simulink model "modello_completo_simulink2019b"  (R2019b)
settings: Solver=VariableStepAuto  StartTime=0.0  StopTime=30  RelTol=1e-3
undefined symbols (not defined in the file): a, a1, a2, AHRS_bias, AHRS_sample_time, AHRS_var, alpha1, alpha2, c, current, D, dead_zone_limit, DiscIntNeverNeededParam, DVL_sample_t, DVL_var1, DVL_var2, DVL_var3, gps_sample_t, H, IMU_sample_time, initial, INSP, Ki_bodypos1, Ki_bodypos2, Ki_bodypos3, Ki_bodypos4, Ki_bodypos5, Ki_depth1, Ki_depth2, Ki_depth3, Ki_depth4, Ki_depth5, Ki_latvel1, Ki_latvel2, Ki_latvel3, Ki_latvel4, Ki_latvel5, Ki_P1, Ki_P2, Ki_P3, Ki_P4, Ki_P5, Ki_R1, Ki_R2, Ki_R3, Ki_R4, Ki_R5, Ki_rel_or1, Ki_rel_or2, Ki_rel_or3, Ki_rel_or4, Ki_rel_or5, Ki_reldist1, Ki_reldist2, Ki_reldist3, Ki_reldist4, Ki_reldist5, Ki_surge1, Ki_surge2, Ki_surge3 ... (+66)
libraries: simulink x3
(part 5 of 5)

== matlab function modello_completo_simulink2019b/Vehicle Model/Thrusters/T/Thruster 7/MATLAB Function ==
  data: n input; T output; V input; D parameter; omega parameter; a1 parameter; a2 parameter; alpha1 parameter; alpha2 parameter
function T = thrusterModel(n, V, D, omega, a1, a2, alpha1, alpha2)

Va = (1-omega) * V;     % Advancement velocity at the propeller
J0 = Va/(n*D);          % Advancement Coefficient

if J0 > -alpha1/alpha2  % Out of linearity domain (right side)
    T = 0;              % A null generated thrust is assumed
    
elseif J0 < 0           % Out of linearity domain (left side)
    T = a1*abs(n)*n;    % Bollard thrust is assumed

else                    % Within the linearity domain
    T = a1*abs(n)*n - a2*abs(n)*V;
end

== matlab function modello_completo_simulink2019b/Vehicle Model/Model Vehicle/MATLAB Function ==
  data: coord_pylon input; eta input; eta_ecef output
function eta_ecef = nedToEcef(coord_pylon, eta)

    coder.extrinsic('wgs84Ellipsoid');

    coder.extrinsic('ned2geodetic');
    
    eta_pos = eta(1:6);
    wgs84 = wgs84Ellipsoid('meter'); %TODO verificare che esprima le coordinate nello stesso modo dell'ECEF dato in missionB.m
    [eta_pos(1), eta_pos(2)] = ned2geodetic(eta(1), eta(2), eta(3), coord_pylon(1), coord_pylon(2), coord_pylon(3), wgs84,'degrees');
    
    eta_pos(3) = eta(3);
    eta_pos(4:6) = eta_pos(4:6);
    
    eta_ecef = eta_pos;
    
end

== matlab function modello_completo_simulink2019b/Vehicle Model/MATLAB Function ==
  data: eta input; ni_c output; current input
function ni_c = current_ned2body(eta, current)
    eta2 = eta(4:6)*pi/180;     % eta2 espresso in radianti
    ni_c = Jac(eta2)'*current;
end

== matlab function modello_completo_simulink2019b/Vehicle Model/Thrusters/T/MATLAB Function ==
  data: ni input; v_th output
function v_th = thrusters(ni)
p1 = [-0.35 -0.25 0]';
p2 = [-0.35 0.25 0]';
p3 = [-0.25 -0.35 0]';
p4 = [0.25 0.35 0]';
p5 = [-0.25 -0.25 -0.19]';
p6 = [-0.25 0.25 -0.19]';
p7 = [0.25 0 -0.19]';

t1 = [1 0 0]';
t2 = t1;
t3 = [0 1 0]';
t4 = -t3;
t5 = [0 0 1]';
t6 = t5;
t7 = t5;

v_lin = ni(1:3);
v_ang = ni(4:6);

vp1 = v_lin + cross(v_ang, p1);
vp2 = v_lin + cross(v_ang, p2);
vp3 = v_lin + cross(v_ang, p3);
vp4 = v_lin + cross(v_ang, p4);
vp5 = v_lin + cross(v_ang, p5);
vp6 = v_lin + cross(v_ang, p6);
vp7 = v_lin + cross(v_ang, p7);

v1 = vp1'*t1;
v2 = vp2'*t2;
v3 = vp3'*t3;
v4 = vp4'*t4;
v5 = vp5'*t5;
v6 = vp6'*t6;
v7 = vp7'*t7;

v_th = [ v1 v2 v3 v4 v5 v6 v7]';
end

== matlab function modello_completo_simulink2019b/Navigation1/Geodetic to NED/MATLAB Function2 ==
  data: GPS_geodetic input; GPS_flag input; GPS_NED output; depth input; pylonCenter parameter
function GPS_NED = Geo2NED(GPS_geodetic, GPS_flag, depth, pylonCenter)

% Funzione che trasforma le coordinate dal sistema di riferimento geodetico
% ad un sistema NED con origine in corrispondenza del centro del pilone.

%% GPS non funzionante
if GPS_flag == 0            
    GPS_NED = [0;0;0];
    return
end

%% Variabili
phi = GPS_geodetic(1);                  % Coordinate geodetiche in radianti                     
lambda = GPS_geodetic(2);  
h = -depth;

phi_pyl = pylonCenter(1) * pi/180;      % Origine del sistema NED in coordinate geodetiche
lambda_pyl = pylonCenter(2) * pi/180;

%% Trasformazione coordinate
coder.extrinsic('wgs84Ellipsoid');
coder.extrinsic('geodetic2ned');
    
[x_gps2, y_gps2, z_gps2] = geodetic2ned(phi, lambda, -depth, phi_pyl, lambda_pyl, 0, wgs84Ellipsoid, 'radians');
eta_NED_GPS = [x_gps2; y_gps2];

GPS_NED = zeros(3,1);
GPS_NED(1) = eta_NED_GPS(1);            % Coordiante NED in radianti
GPS_NED(2) = eta_NED_GPS(2);
GPS_NED(3) = GPS_flag;

== matlab function modello_completo_simulink2019b/Vehicle Model/Thrusters/saturation_tau ==
  data: tau input; tau_sat output; eta input
function tau_sat = sat_tau(tau, eta)
    tau_sat = [0;0;0;0;0;0];
    tau_sat = tau;

    if eta(3) < 0.1 %semiasse c
        tau_sat(3) = 0;
    end
    
end

== matlab function modello_completo_simulink2019b/Navigation1/MATLAB Function1 ==
  data: ang_vel input; DVL input; nu_1 output; c parameter
function nu_1  = dvl2body(ang_vel, DVL, c)

% Funzione che si occupa di trasformare la velocità da sistema di
% riferimento associato al DVL al sistema BODY

% nu_dvl = R_b^dvl (nu_1 + S(nu_2)* P_dvl)
% nu_1 = R_b^dvl' * nu_dvl - S(nu_2) * P_dvl

nu_1    =   zeros(4,1);
nu_2    =   [ang_vel(1); ang_vel(2); ang_vel(3)];
vel_dvl =   [DVL(1); DVL(2); DVL(3)];
R_b_dvl =   eye(3);

S = [   0,          -nu_2(3),   nu_2(2); 
        nu_2(3),    0,          -nu_2(1); 
        -nu_2(2),   nu_2(1),    0       ];
    
p = [0;0;c];

nu_1(1:3) = R_b_dvl' * vel_dvl - S * p;
nu_1(4) = DVL(4); %Flag

== matlab function modello_completo_simulink2019b/Navigation1/MATLAB Function2 ==
  data: Depth_ps input; Depth output; c parameter
function  Depth = ps2body(Depth_ps, c)
% Il profondimetro è posizionato nella parte inferiore dell'AUV, lungo
% l'asse z
Depth = zeros(2,1);
Depth(1) = Depth_ps(1) - c;     %profondità rispetto al centro di massa
Depth(2) = Depth_ps(2);         %flag

== matlab function modello_completo_simulink2019b/Navigation1/AHRS_function ==
  data: eta2 output; lin_acc input; nu2 output; ang_vel input; orientation input
function [eta2, nu2]= AHRS_signals(lin_acc, ang_vel, orientation)
acc = lin_acc(1:3);
nu2 = ang_vel(1:3);
eta2 = orientation(1:3);

== matlab function modello_completo_simulink2019b/Navigation1/DVL_function ==
  data: dvl input; velocity_est output; flag_DVL output
function [velocity_est, flag_DVL] = DVL_signals(dvl)
velocity_est = dvl(1:3);
flag_DVL = dvl(4);

== matlab function modello_completo_simulink2019b/Navigation1/NED to Geodetic/MATLAB Function1 ==
  data: eta_NED input; eta_geodetic output; depth input; pylonCenter parameter
function eta_geodetic = NED2Geo(eta_NED, depth, pylonCenter)

% Funzione che trasforma le coordinate dal sistema NED con origine in
% corrispondenza del centro del pilone al sistema di riferimento geodetico

phi_pyl = pylonCenter(1) * pi/180;      % Origine del sistema NED in coordinate geodetiche 
lambda_pyl = pylonCenter(2) * pi/180;

%% Trasformazione
coder.extrinsic('wgs84Ellipsoid');
coder.extrinsic('ned2geodetic');

[lat, lon, h] = ned2geodetic(eta_NED(1), eta_NED(2), depth, phi_pyl, lambda_pyl, 0, wgs84Ellipsoid, 'radians');

eta_geodetic = [0; 0];
eta_geodetic = [lat; lon];              % Coordiante geodetiche in radianti

== matlab function modello_completo_simulink2019b/Navigation1/Relative estimation/Sonar trigger/MATLAB Function ==
  data: sonar input; sum input; pulse output; prev output
function [pulse, prev] = fcn(sonar, sum)

% La funzione si occupa di monitorare la misura dei sonar,
% quando esse sono modificate manda un impulso al blocco di stima relativa

if nnz(isnan(sum)) > 0 || nnz(sum) == 0 
    pulse = 0;
else
    pulse = 1;
end

prev = sonar;

== matlab function modello_completo_simulink2019b/Navigation1/Relative estimation/Subsystem/MATLAB Function9 ==
  data: sonar input; orientation input; distance output; alpha output; flag_sonar output; pylonRadius parameter; a parameter; s_data parameter
function [distance, alpha, flag_sonar] = relative_values(sonar, orientation, pylonRadius, a, s_data)

% Chiamando la funzione "fcn_sonar" si occupa di calcolate la distanza
% e l'angolo dell'AUV rispetto al pilone

distance = 0;
alpha = 0;
flag_sonar = 0;

coder.extrinsic('fcn_sonar');

[distance, alpha, flag_sonar] = fcn_sonar(sonar, orientation, pylonRadius, a, s_data);
end

== matlab function modello_completo_simulink2019b/Navigation1/flag_function ==
  data: flag_depth input; flag_AHRS input; error_flag output; flag_DVL input; flag_sonar input
function error_flag = fcn(flag_depth, flag_AHRS, flag_DVL, flag_sonar)

% Funzione che rileva la presenza di errore in un sensore

flag_ahrs = flag_AHRS(1) & flag_AHRS(2) & flag_AHRS(3);
error_flag = ~(flag_depth & flag_ahrs & flag_DVL & flag_sonar); % Vale 1 se vi è un errore

== matlab function modello_completo_simulink2019b/Navigation1/z_EKF/EXTENDED KALMAN FILTER/Correzione  ==
  data: prev_pos output; prev_pos input; P input; hat input; meas_pos input; GPS_flag input; meas_depth input; P output; hat output; R parameter; H parameter
function [prev_pos, P, hat] = EKF_pos(prev_pos, P, hat, meas_pos, GPS_flag, meas_depth, R, H)
%% EKF: Correction

% Il filtro corregge i valori di posizione x e y solo quando è disponibile una nuova misura del GPS
if nnz(round(10.^4*(meas_pos - prev_pos))/10.^4) ~= 0 && GPS_flag == 1       % Se il flag è 0 il GPS non funziona

    z_tilde = [ meas_pos(1) - hat(1);
                meas_pos(2) - hat(2);
                meas_depth - hat(3)];

else
        z_tilde = [ 0;
                    0;
                meas_depth - hat(3)];
end
            
    S = H * P * H' + R;

    K = P * H' * S^(-1);
    
    hat = hat + K * z_tilde;
    P = (eye(3) - K * H) * P;  

prev_pos = meas_pos;

== matlab function modello_completo_simulink2019b/Navigation1/z_EKF/EXTENDED KALMAN FILTER/Predizione ==
  data: P input; hat input; dT input; P output; hat output; orientation input; dvl input; ahrs_flag input; init input; P0 input; Q parameter
function [P, hat]  = EKF_pos(P, hat, dT, orientation, dvl, ahrs_flag, init, P0, Q)

dvl_flag = dvl(4);

%% Inizializzazione stato e matrice P
if nnz(hat) == 0           
    hat= init;
    P = P0;
end

if (ahrs_flag && dvl_flag) == 1
    %% Calcolo variabili e matrici
    phi     =   orientation(1);             % roll
    theta   =   orientation(2);             % pitch
    psi_    =   orientation(3);             % yaw
    vel     =   [dvl(1); dvl(2); dvl(3)];  
    
    J       =   zeros(3,3);
    Lk      =   zeros(3,6);
    
    J = [ cos(psi_)*cos(theta), cos(psi_)*sin(phi)*sin(theta) - cos(phi)*sin(psi_), sin(phi)*sin(psi_) + cos(phi)*cos(psi_)*sin(theta);
       cos(theta)*sin(psi_), cos(phi)*cos(psi_) + sin(phi)*sin(psi_)*sin(theta), cos(phi)*sin(psi_)*sin(theta) - cos(psi_)*sin(phi);
         -sin(theta),                                cos(theta)*sin(phi),                                cos(phi)*cos(theta)];
     
    x = dvl(1);
    y = dvl(2);
    z = dvl(3);
    n_ahrs1 = 0;
    n_ahrs2 = 0;
    n_ahrs3 = 0;

    % Matrice Lk: derivata della funzione f rispetto al rumore di AHRS e
    % DVL
    Lk = [  dT*(y*(sin(n_ahrs1 + phi)*sin(n_ahrs3 + psi_) + cos(n_ahrs1 + phi)*cos(n_ahrs3 + psi_)*sin(n_ahrs2 + theta)) + z*(cos(n_ahrs1 + phi)*sin(n_ahrs3 + psi_) - cos(n_ahrs3 + psi_)*sin(n_ahrs1 + phi)*sin(n_ahrs2 + theta))), dT*(z*cos(n_ahrs1 + phi)*cos(n_ahrs3 + psi_)*cos(n_ahrs2 + theta) - x*cos(n_ahrs3 + psi_)*sin(n_ahrs2 + theta) + y*cos(n_ahrs3 + psi_)*cos(n_ahrs2 + theta)*sin(n_ahrs1 + phi)), -dT*(y*(cos(n_ahrs1 + phi)*cos(n_ahrs3 + psi_) + sin(n_ahrs1 + phi)*sin(n_ahrs3 + psi_)*sin(n_ahrs2 + theta)) - z*(cos(n_ahrs3 + psi_)*sin(n_ahrs1 + phi) - cos(n_ahrs1 + phi)*sin(n_ahrs3 + psi_)*sin(n_ahrs2 + theta)) + x*cos(n_ahrs2 + theta)*sin(n_ahrs3 + psi_)), dT*cos(n_ahrs3 + psi_)*cos(n_ahrs2 + theta), -dT*(cos(n_ahrs1 + phi)*sin(n_ahrs3 + psi_) - cos(n_ahrs3 + psi_)*sin(n_ahrs1 + phi)*sin(n_ahrs2 + theta)),  dT*(sin(n_ahrs1 + phi)*sin(n_ahrs3 + psi_) + cos(n_ahrs1 + phi)*cos(n_ahrs3 + psi_)*sin(n_ahrs2 + theta));
     -dT*(y*(cos(n_ahrs3 + psi_)*sin(n_ahrs1 + phi) - cos(n_ahrs1 + phi)*sin(n_ahrs3 + psi_)*sin(n_ahrs2 + theta)) + z*(cos(n_ahrs1 + phi)*cos(n_ahrs3 + psi_) + sin(n_ahrs1 + phi)*sin(n_ahrs3 + psi_)*sin(n_ahrs2 + theta))), dT*(z*cos(n_ahrs1 + phi)*cos(n_ahrs2 + theta)*sin(n_ahrs3 + psi_) - x*sin(n_ahrs3 + psi_)*sin(n_ahrs2 + theta) + y*cos(n_ahrs2 + theta)*sin(n_ahrs1 + phi)*sin(n_ahrs3 + psi_)),  dT*(z*(sin(n_ahrs1 + phi)*sin(n_ahrs3 + psi_) + cos(n_ahrs1 + phi)*cos(n_ahrs3 + psi_)*sin(n_ahrs2 + theta)) - y*(cos(n_ahrs1 + phi)*sin(n_ahrs3 + psi_) - cos(n_ahrs3 + psi_)*sin(n_ahrs1 + phi)*sin(n_ahrs2 + theta)) + x*cos(n_ahrs3 + psi_)*cos(n_ahrs2 + theta)), dT*cos(n_ahrs2 + theta)*sin(n_ahrs3 + psi_),  dT*(cos(n_ahrs1 + phi)*cos(n_ahrs3 + psi_) + sin(n_ahrs1 + phi)*sin(n_ahrs3 + psi_)*sin(n_ahrs2 + theta)), -dT*(cos(n_ahrs3 + psi_)*sin(n_ahrs1 + phi) - cos(n_ahrs1 + phi)*sin(n_ahrs3 + psi_)*sin(n_ahrs2 + theta));
                                                                                                                                    dT*(y*cos(n_ahrs1 + phi)*cos(n_ahrs2 + theta) - z*cos(n_ahrs2 + theta)*sin(n_ahrs1 + phi)),                                                            -dT*(x*cos(n_ahrs2 + theta) + z*cos(n_ahrs1 + phi)*sin(n_ahrs2 + theta) + y*sin(n_ahrs1 + phi)*sin(n_ahrs2 + theta)),                                                                                                                                                                                                                                                                      0,                    -dT*sin(n_ahrs2 + theta),                                                                 dT*cos(n_ahrs2 + theta)*sin(n_ahrs1 + phi),                                                                 dT*cos(n_ahrs1 + phi)*cos(n_ahrs2 + theta)];

    %% EKF: Predizione

    hat  =  hat + dT * J * vel;        
    P =  P + Lk * Q * Lk';            

 
end

== matlab function modello_completo_simulink2019b/Navigation1/z_EKF/Trigger & Init/Depth trigger/MATLAB Function ==
  data: count input; count output; dT output; depth input; sum input; pulse output; prev output
function [count, dT, pulse, prev] = fcn(count, depth, sum)

% La funzione si occupa di monitorare la misura del profondimetro,
% quando essa è modificata manda un impulso al blocco EKF e il tempo
% trascorso dalla precedente variazione

dT = 0;  

if nnz(round(10.^4*sum )/10.^4) == 0
    pulse = 0;
    count = count + 1;
else
    pulse = 1;
    dT = count * (1/200);
    count = 1;
end

prev = depth;

== matlab function modello_completo_simulink2019b/Env. & Sensor Model/GPS SENSOR/NED2Geodetic ==
  data: depth input; u input; data_GDT output; enableGps input; pylonCenter parameter
function data_GDT= fcn(depth, u, enableGps, pylonCenter)

lat_origin = pylonCenter(1);
lon_origin= pylonCenter(2);
h_origin = pylonCenter(3);

xNorth = u(1);
yEast = u(2);

if enableGps==1
    [lat,lon, h] = ned2geodeticS(xNorth, yEast, depth, lat_origin, lon_origin, h_origin);
else
    lat=NaN;
    lon=NaN;
end

data_GDT = [lat, lon];

== matlab function modello_completo_simulink2019b/Env. & Sensor Model/GPS SENSOR/Threshold ==
  data: depth output; x_out output; x_in input; y_out output; y_in input; h_in input; flag_enable_gps output; gpsThreshold parameter
function [depth, x_out, y_out, flag_enable_gps] = fcn(x_in, y_in, h_in, gpsThreshold)


if (h_in > gpsThreshold) % gps does not work
    flag_enable_gps=0;
    x_in = NaN;
    y_in = NaN;
else % ok gps work 
    flag_enable_gps=1;
end

x_out=x_in;
y_out=y_in;
depth=h_in;

== matlab function modello_completo_simulink2019b/Navigation1/z_EKF/Trigger & Init/Initialization/MATLAB Function1 ==
  data: init_counter output; init_counter input; depth input; gps input; GPS_flag input; pulse output; init output; P0 output; prev output; diff_ input; store_gps input; gps_store output; store_depth input; depth_store output; num_cycle parameter
function [init_counter, pulse, init, P0, prev, gps_store, depth_store] = fcn_init(init_counter, depth, gps, GPS_flag, diff_, store_gps, store_depth, num_cycle)

% La funzione si occupa di valutare i valori iniziali dello stato e della varianza dell'errore di stima

%% Variabili
pulse = 0;
gps_store = store_gps;
depth_store = store_depth;
init = zeros(3,1);
P0 = zeros(3);
coder.extrinsic('init_position');

%%
if nnz(round(10.^4*diff_)/10.^4) ~= 0 && init_counter < num_cycle && GPS_flag == 1
    
    init_counter = init_counter + 1;
    gps_store(1, init_counter) = gps(1);
    gps_store(2, init_counter) = gps(2);
    pulse = 0;
    depth_store(init_counter) = depth;

        
elseif init_counter < num_cycle

    init_counter = init_counter;
    pulse = 0;
    
    
elseif init_counter >= num_cycle && init_counter < 300
   
    [init, P0] = init_position(store_gps, store_depth, num_cycle); 
    pulse = 1;
    init_counter = init_counter + 1;

else 
    
    pulse = 1;
   
end

prev = gps;

== matlab function modello_completo_simulink2019b/Env. & Sensor Model/AHRS SENSOR/    ==
  data: ni_1 input; ni_1_dot input; lin_acc output; ang_vel output; m output; ni_2 input; eta_2 input; eta_2_dot input
function [lin_acc, ang_vel, m] = IMU(ni_1, ni_1_dot, ni_2, eta_2, eta_2_dot)

% questa funzione, partendo dalle informazioni cinematiche dell' AUV
% restituisce in output delle misure di accelerazione, velocità angolare
% e campo magnetico locale


% definisco R^T
% R = Rz(psi)*Ry(theta)*Rx(phi);

% yaw = psi; pitch = theta; roll = phi;

phi = eta_2(1);
theta = eta_2(2);
psi = eta_2(3);

R = [cos(psi)*cos(theta) cos(psi)*sin(theta)*sin(phi)-sin(psi)*cos(phi) cos(psi)*sin(theta)*cos(phi)+sin(psi)*sin(phi);
     sin(psi)*cos(theta) sin(psi)*sin(theta)*sin(phi)+cos(psi)*cos(phi) sin(psi)*sin(theta)*cos(phi)-cos(psi)*sin(phi);
    -sin(theta) cos(theta)*sin(phi) cos(theta)*cos(phi)];

% Rx_phi = [1 0 0; 0 cos(phi) sin(phi); 0 -sin(phi) cos(phi)];
% Ry_theta = [cos(theta) 0 -sin(theta); 0 1 0; sin(theta) 0 cos(theta)];
% Rz_psi = [cos(psi) sin(psi) 0; -sin(psi) cos(psi) 0; 0 0 1];

% R = Rz_psi'*Ry_theta'*Rx_phi;

% Definisco la matrice Jacobiana
 
%J_2 = [1 sin(phi)*tan(theta) cos(phi)*tan(theta);
%       0 cos(phi) -sin(phi);
%       0 sin(phi)/cos(theta) cos(phi)/cos(theta)];
  
% accelerometro

g = [0 0 9.82]; % [m/s^2]
 
%lin_acc = J_1' * (eta_1_ddot - g);  
 
% eta_1_ddot = J_1 * ni_1_dot + J_1_dot * ni_1

dphi = eta_2_dot(1);
dtheta = eta_2_dot(2);
dpsi = eta_2_dot(3);


J_1_dot = [-dtheta*(sin(theta)*cos(psi)) - dpsi*(sin(psi)*cos(theta)), ...
           dphi*(sin(psi)*sin(phi) + cos(psi)*sin(theta)*cos(phi)) + dtheta*(cos(psi)*cos(theta)*sin(phi)) - dpsi*(cos(psi)*cos(phi) + sin(psi)*sin(theta)*sin(phi)), ... 
           dphi*(sin(psi)*cos(phi) - cos(psi)*sin(theta)*sin(phi)) + dtheta*(cos(psi)*cos(theta)*cos(phi)) + dpsi*(cos(psi)*sin(phi) - sin(psi)*sin(theta)*cos(phi)); ...
          -dtheta*(sin(theta)*sin(psi)) + dpsi*(cos(psi)*cos(theta)), ...
           dphi*(-cos(psi)*sin(phi) + sin(psi)*sin(theta)*cos(phi)) + dtheta*(sin(psi)*cos(theta)*sin(phi)) + dpsi*(-sin(psi)*cos(phi) + cos(psi)*sin(theta)*sin(phi)), ... 
          -dphi*(cos(psi)*cos(phi) + sin(psi)*sin(theta)*sin(phi)) + dtheta*(sin(psi)*cos(theta)*cos(phi)) + dpsi*(sin(psi)*sin(phi) + cos(psi)*sin(theta)*cos(phi)); ...
          -dtheta*(cos(theta)), ...
           dphi*(cos(theta)*cos(phi)) - dtheta*(sin(theta)*sin(phi)), ...
          -dphi*(cos(theta)*sin(phi)) - dtheta*(sin(theta)*cos(phi))];

% J_1 = R;      

eta_1_ddot = R * ni_1_dot + J_1_dot * ni_1;

lin_acc = R' * (eta_1_ddot - g');
 
 
 %  giroscopio
 
 % se mi fosse stata fornita la eta_2_dot (espressa in terna NED, globale) la
 % misura del giroscopio sarebbe stata:
 
 %ang_vel = inv(J_2) * eta_2_dot;
 
 %avendo a disposizione in ingresso l'accelerazione in terna Body, la
 %misura della velocità angolare sarà:
 
 ang_vel = ni_2;
 
 % magnetometro ( campo magnetico terrestre espresso in terna NED)
 
 
% gaussian =  normrnd([0 0 0], [0.00131, 0.00094, 0.00157]);
% gaussian = incertezza dell'intensità del campo magnetico 
% calcolata su: https://www.ngdc.noaa.gov/geomag/calculators/magcalc.shtml#igrfwmm

 m_e = [0.238836 -0.010851 0.392423]'; % + gaussian';
 
 m = R' * m_e;
 
end

== matlab function modello_completo_simulink2019b/Env. & Sensor Model/DVL SENSOR/MATLAB Function ==
  data: ni input; niDVL output; c parameter
function niDVL = traslation(ni, c)
%Calcola la velocità in terna DVL

S = [0,-ni(6),ni(5); 
    ni(6),0,-ni(4); 
    -ni(5),ni(4),0];
p = [0;0;c];
niDVL = ni(1:3,1)+S*p;        %Formula fondamentale della cinematica

== matlab function modello_completo_simulink2019b/Env. & Sensor Model/DVL SENSOR/MATLAB Function2 ==
  data: v input; flag output
function flag  = vel_module(v)
%Calcola il modulo della velocità per controllare le condizioni di
%funzionamento del DVL

mod = sqrt((v(1))^2+(v(2))^2+(v(3))^2);

%Da datasheet, se la velocità è superiore ai 9 m/s il sensore non funziona bene
if mod > 9
    flag = 0;
else
    flag = 1;
end
end

== matlab function modello_completo_simulink2019b/Controller/AVVICINAMENTO/J2_inv ==
  data: tau_roll input; tau_or_body output; tau_pitch input; tau_yaw input; est_state input
function tau_or_body = fcn(tau_roll,tau_pitch,tau_yaw,est_state)
theta=est_state(1);
phi=est_state(2);
tau_or=[tau_roll;tau_pitch;tau_yaw];
J2_inv = [1       0          -sin(theta); 
         0   cos(phi)  cos(theta)*sin(phi);
         0  -sin(phi)  cos(theta)*cos(phi)];
tau_or_body=J2_inv*tau_or;
end

== matlab function modello_completo_simulink2019b/Controller/GEODETIC2NED2/GEODETIC2NED1/MATLAB Function ==
  data: lat input; pos_s_Ned output; lon input
function pos_s_Ned = fcn(lat,lon)
coder.extrinsic('wgs84Ellipsoid','geodetic2ned');
pylonCenter = [43.723046;10.396635];
initPoint = [ 43.722984;10.396204;0];
hOrigin=0;
pos_s_Ned=zeros(3,1);
wgs84=wgs84Ellipsoid('meter');
lat0=pylonCenter(1);
lon0=pylonCenter(2);
h=initPoint(3);
h0=hOrigin;
[xs_N,ys_E,zs_D]=geodetic2ned(lat,lon,h,lat0,lon0,h0,wgs84);
pos_s_Ned=[xs_N,ys_E,zs_D]';
end

== matlab function modello_completo_simulink2019b/Env. & Sensor Model/Pressure sensor/MATLAB Function2 ==
  data: h input; p output; rho parameter
function p = pressure(h, rho)
%Calcola la pressione a partire dalla profondità

g = 9.81;                        %accelerazione gravitazionale
p = rho*g*h;
end

== matlab function modello_completo_simulink2019b/Env. & Sensor Model/Pressure sensor/MATLAB Function3 ==
  data: orient input; p input; h output; rho parameter; c parameter
function h = depth( orient,  p, rho, c)
%Calcola la profondità misurata dal sensore

phi = orient(1);
theta = orient(2);
psi = orient(3);
Rx_phi = [1 0 0; 0 cos(phi) -sin(phi); 0 sin(phi) cos(phi)];
Ry_theta = [cos(theta) 0 sin(theta); 0 1 0; -sin(theta) 0 cos(theta)];
Rz_psi = [cos(psi) -sin(psi) 0; sin(psi) cos(psi) 0; 0 0 1];

R = Rz_psi*Ry_theta*Rx_phi;
g = 9.81;
cNED = R*[0;0;c];                            %Vettore posizione dell'AUV in terna body riportato in terna NED
h = p/(rho*g)+cNED(3);                       %Il profondimetro è installato sulla pancia dell'AUV, lungo l'asse z
end

== matlab function modello_completo_simulink2019b/Controller/GEODETIC2NED3/GEODETIC2NED/MATLAB Function ==
  data: lat input; lon input; pos_Ned output
function pos_Ned = fcn (lat,lon)
coder.extrinsic('wgs84Ellipsoid','geodetic2ned');
pylonCenter = [43.723046;10.396635];
initPoint = [ 43.722984;10.396204;0];
hOrigin=0;
pos_Ned=zeros(3,1);
wgs84=wgs84Ellipsoid('meter');
h=initPoint(3);
lat0=pylonCenter(1);
lon0=pylonCenter(2);
h0=hOrigin;
[x_N,y_E,z_D]=geodetic2ned(lat,lon,h,lat0,lon0,h0,wgs84);
pos_Ned=[x_N,y_E,z_D]';
end

== matlab function modello_completo_simulink2019b/Controller/IMMERSIONE//RISALITA/J2_inv ==
  data: tau_roll input; tau_or_body output; tau_pitch input; tau_yaw input; est_state input
function tau_or_body = fcn(tau_roll,tau_pitch,tau_yaw,est_state)
theta=est_state(1);
phi=est_state(2);
tau_or=[tau_roll;tau_pitch;tau_yaw];
J2_inv = [1       0          -sin(theta); 
         0   cos(phi)  cos(theta)*sin(phi);
         0  -sin(phi)  cos(theta)*cos(phi)];
tau_or_body=J2_inv*tau_or;
end

== matlab function modello_completo_simulink2019b/Env. & Sensor Model/Sonar sensor/MATLAB Function ==
  data: xNorth input; s output; yEast input; zDown input; roll input; pitch input; yaw input; pylonRadius parameter; s_data parameter
function s = Sonar_ideal(xNorth,yEast,zDown,roll,pitch,yaw,pylonRadius, s_data)

coder.extrinsic('Sonar_id');

s_data.num = 5;
s = zeros(s_data.num,1);

s = Sonar_id(xNorth,yEast,zDown,roll,pitch,yaw,pylonRadius,s_data);

== matlab function modello_completo_simulink2019b/Env. & Sensor Model/Sonar sensor/MATLAB Function1 ==
  data: s_in input; s_out output; depth input; error input; flag output; s_data parameter
function [s_out,flag] = Sonar_lim(s_in,depth,error,s_data)
%SONAR_lim
%     [s_out,flag] = Sonar_id[s,error]
%
% Returns the sonar output considering the sensors limitations, but not
% taking into account the bias and error.
%
% flag signals that the corresponding sensor output is affected by
% problems:
% flag += 0     ==>     No errors
% flag += 1     ==>     Under minimum detectable range
% flag += 2     ==>     Over maximum detectable range
% flag += 4     ==>     Over maximum depth
% flag += 8     ==>     Other errors
%
% error is a boolean variable which, when true, sets the flag to += 8

s_data.num = 5;

flag = zeros(s_data.num,1);

s_out = s_in;

for i=1:s_data.num
    if s_in(i) < s_data.minrng
    % Too close
        flag(i) = flag(i)+1;
        s_out(i) = s_data.minrng;
    end
    
    if ( s_in(i) > s_data.maxrng || isnan(s_in(i)) )
    % Too far
        flag(i) = flag(i)+2;
        s_out(i) = NaN;
    end
    
    if depth > s_data.maxdpt
    % Over max depth
        flag(i) = flag(i)+4;
        s_out(i) = NaN;
    end
    
    if error(i) > 0
    % General error flag
        flag(i) = flag(i) + error(i);
        s_out(i) = NaN;
    end
end

end

== matlab function modello_completo_simulink2019b/Controller/MATLAB Function1 ==
  data: STATE input; EN output; bodyposx_err input; yaw_err input; depth_err input; INSP input string
function EN = fcn(STATE,bodyposx_err,yaw_err,depth_err, INSP)

%EN(1)= bodypos_err
%EN(2)= rel_dist_err
%EN(3)=surge_err
%EN(4)= latvel_err
%EN(5)=depth_err
%EN(6)= RP_err
%EN(7)= rel_or_err
%EN(8)= yaw_err

EN=zeros(1,8)';

if (STATE == 101)
    EN(8)=1;
end
%avvicinamento pilone
if (STATE== 102)
    EN(8)=1;
    EN(3)=1;
    if (STATE==102) && (bodyposx_err<=3)
        EN(8)=1;
        EN(1)=1;
        EN(3)=0;
    end
end
%rotazione attorno al pilone in superficie
if (STATE == 103)
    EN(2)=1;
    EN(7)=1;
    EN(4)=1;    
    if (yaw_err<=10)
        EN(4)=0;
        EN(8)=1;
        EN(2)=1;
        EN(7)=0;
    end
end
%unicodestr = native2unicode(INSP);
s1=INSP;
s2='vertical';
CMP=strcmp(s1,s2);
if (CMP == 1) %inizio ispezione verticale
    if (STATE==201) 
        EN(2)=1;
        EN(5)=1;
        EN(7)=1;
        EN(6)=1;
        if(depth_err<=3) %stacco i thrusters che controllano la depth
            EN(2)=1;
            EN(7)=1;
            EN(5)=0;
            EN(6)=1;   
        end
    end
    if(STATE==202) && (depth_err<0.2) %controllo di velocità laterale
        EN(2)=1;
        EN(4)=1;
        EN(5)=1;
        EN(6)=1;
        EN(7)=1;
        if(yaw_err<=10) %switch su controllo di posizione
            EN(8)=1;
            EN(2)=1;
            EN(7)=0;
            EN(4)=0; 
            EN(5)=1;
            EN(6)=1;
        end
    end  %fine ispezione verticale
else
    if (STATE==202) && (depth_err<0.2) % inizio ispezione orizzontale
        EN(2)=1;
        EN(5)=1;
        EN(4)=1;  
        EN(7)=1;  
        EN(6)=1;
        if(yaw_err<=10) %switch su controllo di yaw
            EN(8)=1;
            EN(2)=1;
            EN(7)=0; 
            EN(4)=0;
            EN(5)=1;
            EN(6)=1;
        end
    end
    if (STATE==201) %transetto verticale in isp. orizzontale
        EN(2)=1;
        EN(7)=1;
        EN(5)=1;
        EN(6)=1;   
    end 
end     %fine ispezione orizzontale
%fase di immersione   
if(STATE==104)
   EN(2)=1;
   EN(7)=1;
   EN(5)=1;
   EN(6)=1;
   if(depth_err<=3) %stacco i thrusters che controllano la depth
        EN(2)=1;
        EN(7)=1;
        EN(5)=0;
        EN(6)=1;   
   end
end
%fase di risalita
if(STATE==401)
   EN(2)=1;
   EN(7)=1;
   EN(5)=1;
   EN(6)=1;
end   
   
%fase di errore e fine missione
if(STATE == 500) || (STATE == 999)% lascio così poichè in caso di errore
   EN=zeros(1,8)';               % comunque spegnamo tutti i segnali e
                                % lo facciamo risalire attraverso i 4N
end
end

== matlab function modello_completo_simulink2019b/Env. & Sensor Model/geodetic2NED1 ==
  data: x output; u input; y output; z output; pylonCenter parameter
function [x, y, z] = fcn(u, pylonCenter)


lat_origin = pylonCenter(1);
lon_origin= pylonCenter(2);
h_origin = pylonCenter(3);

lat=u(1);
lon=u(2);
h=u(3);


[xNorth, yEast, zDown] = geodetic2nedS(lat, lon, h, lat_origin, lon_origin, h_origin);

x = xNorth;
y = yEast;
z = h;

== matlab function modello_completo_simulink2019b/Controller/NED2BODY ==
  data: eta1_dot input; mi1 output; phi input; theta input; psi input
function mi1 = fcn(eta1_dot,phi,theta,psi)
Rx_phi=[1 0 0;0 cos(phi) -sin(phi);0 sin(phi) cos(phi)];
Ry_theta=[cos(theta) 0 sin(theta);0 1 0;-sin(theta) 0 cos(theta)];
Rz_psi=[cos(psi) -sin(psi) 0;sin(psi) cos(psi) 0;0 0 1];
J1=Rx_phi*Ry_theta*Rz_psi;
mi1 =J1^-1*eta1_dot;

== matlab function modello_completo_simulink2019b/Controller/NED2BODY1 ==
  data: abspos_err input; bodypos_err output; phi input; theta input; psi input
function bodypos_err = fcn(abspos_err,phi,theta,psi)
Rx_phi=   [1      0        0;
           0   cos(phi) -sin(phi);
           0   sin(phi) cos(phi)];
    
Ry_theta=[cos(theta) 0  sin(theta);
              0      1      0;
         -sin(theta) 0  cos(theta)];
     
Rz_psi=  [cos(psi) -sin(psi)  0;
          sin(psi)  cos(psi)  0;
           0           0      1];
       
J1=Rx_phi*Ry_theta*Rz_psi;
bodypos_err=J1^-1*abspos_err;

== matlab function modello_completo_simulink2019b/Controller/POSIZIONAMENTO/J2_inv ==
  data: tau_roll input; tau_or_body output; tau_pitch input; tau_yaw input; est_state input
function tau_or_body = fcn(tau_roll,tau_pitch,tau_yaw,est_state)
theta=est_state(1);
phi=est_state(2);
tau_or=[tau_roll;tau_pitch;tau_yaw];
J2_inv = [1       0          -sin(theta); 
         0   cos(phi)  cos(theta)*sin(phi);
         0  -sin(phi)  cos(theta)*cos(phi)];
tau_or_body=J2_inv*tau_or;
end

== matlab function modello_completo_simulink2019b/Controller/ROTAZIONE IN PROFONDITA'/J2_inv ==
  data: tau_roll input; tau_or_body output; tau_pitch input; tau_yaw input; est_state input
function tau_or_body = fcn(tau_roll,tau_pitch,tau_yaw,est_state)
theta=est_state(1);
phi=est_state(2);
tau_or=[tau_roll;tau_pitch;tau_yaw];
J2_inv = [1       0          -sin(theta); 
         0   cos(phi)  cos(theta)*sin(phi);
         0  -sin(phi)  cos(theta)*cos(phi)];
tau_or_body=J2_inv*tau_or;
end

== matlab function modello_completo_simulink2019b/Controller/ROTAZIONE IN SUPERFICIE/J2_inv ==
  data: tau_roll input; tau_or_body output; tau_pitch input; tau_yaw input; est_state input
function tau_or_body = fcn(tau_roll,tau_pitch,tau_yaw,est_state)
theta=est_state(1);
phi=est_state(2);
tau_or=[tau_roll;tau_pitch;tau_yaw];
J2_inv = [1       0          -sin(theta); 
         0   cos(phi)  cos(theta)*sin(phi);
         0  -sin(phi)  cos(theta)*cos(phi)];
tau_or_body=J2_inv*tau_or;
end

== matlab function modello_completo_simulink2019b/Controller/T2n/MATLAB Function ==
  data: Tdes input; n output
function n  = fcn(Tdes)
n=zeros(1,7)';
a1=0.000388302366464000;
%assunzione modello a bassa velocità
for i=1:1:7
       n(i)=sign(Tdes(i))*sqrt((abs(Tdes(i))/a1));  
end
end

== matlab function modello_completo_simulink2019b/Controller/Tau2T/Tau2T ==
  data: tau_des input; T output
function T= fcn(tau_des)
p1 = [0 -0.25 0]';
p2 = [0 0.25 0]';
p3 = [-0.25 0 0]';
p4 = [0.25 0 0]';
p5 = [-0.15 -0.15 0]';
p6 = [-0.15 0.15 0]';
p7 = [0.15 0 0]';

t1 = [1 0 0]';
t2 = t1;
t3 = [0 1 0]';
t4 = -t3;
t5 = [0 0 1]';
t6 = t5;
t7 = t5;

B1 = [t1; cross(p1,t1)];
B2 = [t2; cross(p2,t2)];
B3 = [t3; cross(p3,t3)];
B4 = [t4; cross(p4,t4)];
B5 = [t5; cross(p5,t5)];
B6 = [t6; cross(p6,t6)];
B7 = [t7; cross(p7,t7)];
B = [B1 B2 B3 B4 B5 B6 B7];

Bpinv=pinv(B);
T = Bpinv*tau_des;

end

== matlab function modello_completo_simulink2019b/Controller/Tau2T/Tau_des ENABLE ==
  data: STATE input; tau_des output; tau1 input; tau2 input; tau3 input; tau4 input; tau5 input
function tau_des= fcn(STATE,tau1,tau2,tau3,tau4,tau5)
tau_des= zeros(1,6)';
if (STATE==101)
    tau_des=tau1;
end
if (STATE==102)
    tau_des=tau2;
end
if (STATE==103)
    tau_des= tau3;
end
if (STATE== 201|| STATE==104||STATE==401)
    tau_des=tau4;
end
if (STATE== 202)
    tau_des=tau5;
end
if (STATE==500 || STATE== 999)
    tau_des=zeros(1,6)';
end
end

== matlab function modello_completo_simulink2019b/Controller/wrapTopi ==
  data: u input; y output
function y = fcn(u)
coder.extrinsic('wrapToPi');
y=0;
y = wrapToPi(u);
end

== matlab function modello_completo_simulink2019b/Controller/wrapTopi1 ==
  data: u input; y output
function y = fcn(u)
coder.extrinsic('wrapToPi');
y=0;
y = wrapToPi(u);
end

== matlab function modello_completo_simulink2019b/Navigation1/Relative estimation/flag_sonar_func ==
  data: flag_sonar input; flag output; s_data parameter
function flag = fcn(flag_sonar, s_data)

flag = 1;

if sum(flag_sonar) >= (s_data.num-1)*8
    flag = 0;
else 
    flag = 1;
end
